simulink model "P_2_1_j_Forditott_inga_egyensulyozasa_kocsin"  (R2021b)
settings: Solver=ode5  StartTime=0.0  StopTime=10  FixedStep=0.01  RelTol=1e-3
model workspace (MAT data in the model file):
  M = Simulink.Signal
  M.DataType = 'auto'
  M.Dimensions = -1
  M.DimensionsMode = 'auto'
  M.Complexity = 'auto'
  M.SampleTime = -1
  M.SamplingMode = 'auto'
  g = Simulink.Signal
  g.DataType = 'auto'
  g.Dimensions = -1
  g.DimensionsMode = 'auto'
  g.Complexity = 'auto'
  g.SampleTime = -1
  g.SamplingMode = 'auto'
  l = Simulink.Signal
  l.DataType = 'auto'
  l.Dimensions = -1
  l.DimensionsMode = 'auto'
  l.Complexity = 'auto'
  l.SampleTime = -1
  l.SamplingMode = 'auto'
  m = Simulink.Signal
  m.DataType = 'auto'
  m.Dimensions = -1
  m.DimensionsMode = 'auto'
  m.Complexity = 'auto'
  m.SampleTime = -1
  m.SamplingMode = 'auto'
settings Model: Creator=davidpaksi  LastModifiedBy=davidpaksi

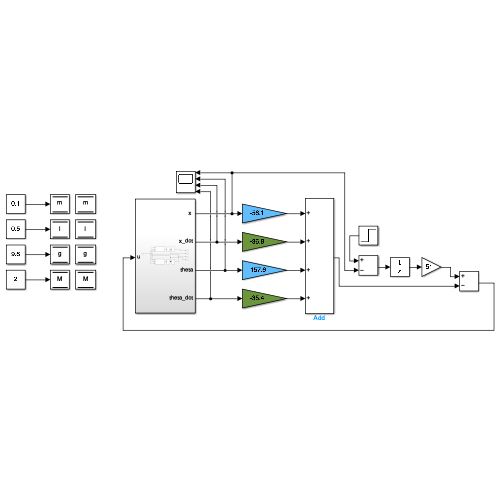
[thumbnail: Simulink's stored preview of the top-level diagram]
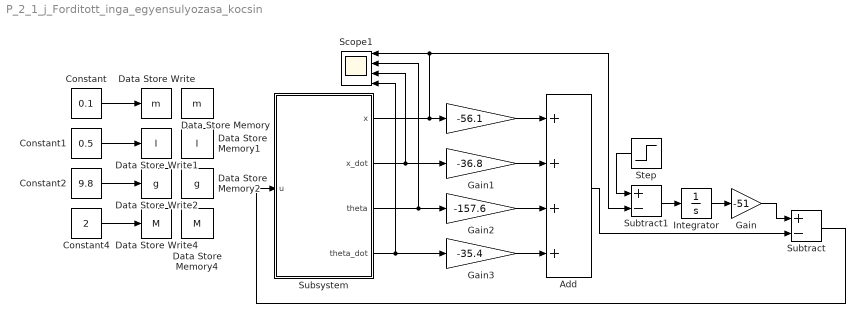
== system P_2_1_j_Forditott_inga_egyensulyozasa_kocsin ==
  " " : Gain  Gain=-56.1
  Add : Sum  Inputs=++++
  Constant : Constant  Value=0.1
  Constant1 : Constant  Value=0.5
  Constant2 : Constant  Value=9.8
  Constant4 : Constant  Value=2
  Data Store Memory : DataStoreMemory  DataStoreName=m  ReadBeforeWriteMsg=warning  WriteAfterWriteMsg=warning  WriteAfterReadMsg=warning  ShowAdditionalParam=off  OutDataTypeStr=double  StateMustResolveToSignalObject=on
  Data Store Memory1 : DataStoreMemory  DataStoreName=l  ReadBeforeWriteMsg=warning  WriteAfterWriteMsg=warning  WriteAfterReadMsg=warning  ShowAdditionalParam=off  OutDataTypeStr=double  StateMustResolveToSignalObject=on
  Data Store Memory2 : DataStoreMemory  DataStoreName=g  ReadBeforeWriteMsg=warning  WriteAfterWriteMsg=warning  WriteAfterReadMsg=warning  ShowAdditionalParam=off  OutDataTypeStr=double  StateMustResolveToSignalObject=on
  Data Store Memory4 : DataStoreMemory  DataStoreName=M  ReadBeforeWriteMsg=warning  WriteAfterWriteMsg=warning  WriteAfterReadMsg=warning  ShowAdditionalParam=off  OutDataTypeStr=double  StateMustResolveToSignalObject=on
  Data Store Write : DataStoreWrite  DataStoreName=m  IndexOptions=Index vector (dialog)  Indices=1  OutputSizes=1
  Data Store Write1 : DataStoreWrite  DataStoreName=l  IndexOptions=Index vector (dialog)  Indices=1  OutputSizes=1
  Data Store Write2 : DataStoreWrite  DataStoreName=g  IndexOptions=Index vector (dialog)  Indices=1  OutputSizes=1
  Data Store Write4 : DataStoreWrite  DataStoreName=M  IndexOptions=Index vector (dialog)  Indices=1  OutputSizes=1
  Gain : Gain  Gain=-51
  Gain1 : Gain  Gain=-36.8
  Gain2 : Gain  Gain=-157.6
  Gain3 : Gain  Gain=-35.4
  Integrator : Integrator
  Scope1 : Scope  NumInputPorts=4
  Step : Step  After=2
  Subsystem : Subsystem
  Subtract : Sum  Inputs=+-
  Subtract1 : Sum  Inputs=+-
  wires:
  Constant/1 -> Data Store Write/1
  Constant1/1 -> Data Store Write1/1
  Constant2/1 -> Data Store Write2/1
  Constant4/1 -> Data Store Write4/1
  Add/1 -> Subtract/2
  Subtract1/1 -> Integrator/1
  Integrator/1 -> Gain/1
  Step/1 -> Subtract1/1
  Subtract/1 -> Subsystem/1(u)
  Subsystem/1(" x ") -> Scope1/1, Subtract1/2, " "/1
  " "/1 -> Add/1
  Gain1/1 -> Add/2
  Subsystem/2(" x_dot") -> Gain1/1, Scope1/3
  Subsystem/3(" theta") -> Gain2/1, Scope1/2
  Gain2/1 -> Add/3
  Gain3/1 -> Add/4
  Subsystem/4(" theta_dot") -> Scope1/4, Gain3/1
  Gain/1 -> Subtract/1

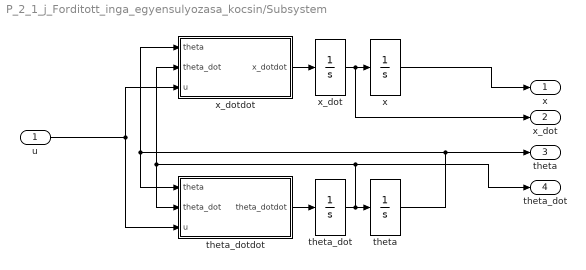
== system P_2_1_j_Forditott_inga_egyensulyozasa_kocsin/Subsystem ==
  u : Inport
  theta : Integrator
  theta_dot : Integrator
  theta_dotdot : MATLAB Function  TreatAsAtomicUnit=on
  x : Integrator
  x_dot : Integrator
  x_dotdot : MATLAB Function  TreatAsAtomicUnit=on
  " x " : Outport
  " x_dot" : Outport  Port=2
  " theta" : Outport  Port=3
  " theta_dot" : Outport  Port=4
  wires:
  x_dotdot/1(x_dotdot) -> x_dot/1
  theta_dotdot/1(theta_dotdot) -> theta_dot/1
  u/1 -> x_dotdot/3(u), theta_dotdot/3(u)
  x_dot/1 -> " x_dot"/1, x/1
  theta/1 -> " theta"/1, x_dotdot/1(theta), theta_dotdot/1(theta)
  theta_dot/1 -> " theta_dot"/1, x_dotdot/2(theta_dot), theta_dotdot/2(theta_dot), theta/1
  x/1 -> " x "/1

== matlab function P_2_1_j_Forditott_inga_egyensulyozasa_kocsin/Subsystem/theta_dotdot ==
  settings: updateMethod=DISCRETE
  data: theta input; theta_dotdot output; theta_dot input; m data_store_memory; l data_store_memory; g data_store_memory; M data_store_memory; u input
function theta_dotdot = fcn(theta,theta_dot,u)
global m l g M
theta_dotdot = -(m*l*theta_dot^2*sin(theta)*cos(theta)-m*g*sin(theta)+u*cos(theta)-M*g*sin(theta))/(l*(M+m*sin(theta)^2));
%              -(cos(u(5))*sin(u(5))*m*l*u(4)*u(4)-m*g*sin(u(5))+u(3)*cos(u(5))-g*M*sin(u(5)))/(l*(M+m*sin(u(5))*sin(u(5))))

== matlab function P_2_1_j_Forditott_inga_egyensulyozasa_kocsin/Subsystem/x_dotdot ==
  settings: updateMethod=DISCRETE
  data: theta input; x_dotdot output; theta_dot input; m data_store_memory; l data_store_memory; g data_store_memory; M data_store_memory; u input
function x_dotdot = fcn(theta, theta_dot, u)
